simulink model "ex4_3"  (R2017a)
settings: Solver=ode23t  StartTime=0.0  StopTime=.3  MaxStep=1e-5  RelTol=1e-4  EnableMultiTasking=on
undefined symbols (not defined in the file): jsin
libraries: simulink x1, powerlib x1
settings Model: Creator=hi  LastModifiedBy=Omid
settings DataIOCC: LimitDataPoints=on
settings OptimizationCC: LifeSpan=inf
settings DebuggingCC: SFUnexpectedBacktrackingDiag=warning  SFNoUnconditionalDefaultTransitionDiag=warning  SFExecutionAtInitializationDiag=none
settings HardwareCC: ProdBitPerSizeT=32  ProdBitPerPtrDiffT=32  ProdWordSize=32  ProdHWDeviceType=Specified
settings ModelReferenceCC: PropagateSignalLabelsOutOfModel=off
settings GRTTargetCC: TargetLangStandard=C89/C90 (ANSI)
settings ConfigComp: CovMetricSettings=dw  CovSaveCumulativeToWorkspaceVar=on  CovSaveSingleToWorkspaceVar=on  CovExternalEMLEnable=off
settings SimscapeCC: SimscapeNormalizeSystem=off
settings ConfigurationSet: Description=SimMechanics 2G

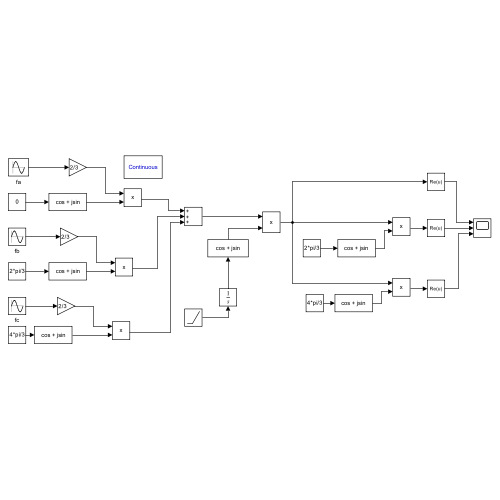
[thumbnail: Simulink's stored preview of the top-level diagram]
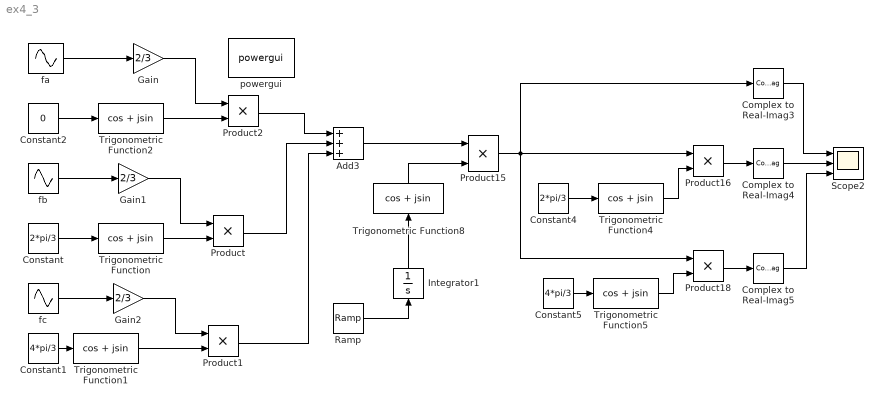
== system ex4_3 ==
  Add3 : Sum  Inputs=+++
  Complex to Real-Imag3 : ComplexToRealImag  Output=Real
  Complex to Real-Imag4 : ComplexToRealImag  Output=Real
  Complex to Real-Imag5 : ComplexToRealImag  Output=Real
  Constant : Constant  Value=2*pi/3
  Constant1 : Constant  Value=4*pi/3
  Constant2 : Constant  Value=0
  Constant4 : Constant  Value=2*pi/3
  Constant5 : Constant  Value=4*pi/3
  Gain : Gain  Gain=2/3
  Gain1 : Gain  Gain=2/3
  Gain2 : Gain  Gain=2/3
  Integrator1 : Integrator
  Product{,1..2,15..16,18} (6 alike) : Product
  Ramp : simulink/Sources/Ramp  slope=-2*pi*400  start=0  X0=0
  Scope2 : Scope  NumInputPorts=3
  Trigonometric Function{,1..2,4..5,8} (6 alike) : Trigonometry  Operator=cos + jsin
  fa : Sin  Frequency=377  Phase=pi/2  SampleTime=0
  fb : Sin  Frequency=377  Phase=-2*pi/3+pi/2  SampleTime=0
  fc : Sin  Frequency=377  Phase=-4*pi/3+pi/2  SampleTime=0
  powergui : powerlib/powergui  Priority=1  SimulationMode=Continuous  SampleTime=50e-6  frequency=60  Iterations=50  frequencyindice=60  Pbase=100e6  ErrMax=1e-4  UnitsV=kV  UnitsW=MW  buscounter=0  FunctionMessages=off  echomessages=off  EnableUseOfTLC=off  CurrentSourceSwitches=on  DisableSnubberDevices=off  DisableRonSwitches=off  DisableVfSwitches=off  DisplayEquations=off  AutomaticDiscreteSolvers=off  SolverType=Tustin/Backward Euler (TBE)  Interpol=off  ExternalGateDelay=off  methode=off  Ts=10  x0status=blocks  SPID=off  SwTol=0  HookPort=off  NonlinearTolerance=1e-4  nMaxIteration=100  ContinueOnMaxIteration=off  RestoreLinks=warning  ResistiveCurrentMeasurement=off  Frange=[0:2:500]  Ylog=off  Xlog=on  ShowGrid=off  save=off  variable=ZData  structure=0  ZoomFFT=off  StartTime=0.0  cycles=1  DisplayStyle=1  fundamental=60  FreqAxis=off  MaxFrequency=1000  frequencyindicesteady=1  RmsSteady=1  display=off
  wires:
  Constant/1 -> Trigonometric Function/1
  Trigonometric Function/1 -> Product/2
  Trigonometric Function1/1 -> Product1/2
  Constant1/1 -> Trigonometric Function1/1
  fc/1 -> Gain2/1
  fb/1 -> Gain1/1
  Constant2/1 -> Trigonometric Function2/1
  Trigonometric Function2/1 -> Product2/2
  fa/1 -> Gain/1
  Product2/1 -> Add3/1
  Product/1 -> Add3/2
  Product1/1 -> Add3/3
  Add3/1 -> Product15/1
  Constant4/1 -> Trigonometric Function4/1
  Constant5/1 -> Trigonometric Function5/1
  Product15/1 -> Complex to Real-Imag3/1, Product16/1, Product18/1
  Trigonometric Function4/1 -> Product16/2
  Trigonometric Function5/1 -> Product18/2
  Product16/1 -> Complex to Real-Imag4/1
  Product18/1 -> Complex to Real-Imag5/1
  Complex to Real-Imag4/1 -> Scope2/2
  Complex to Real-Imag3/1 -> Scope2/1
  Complex to Real-Imag5/1 -> Scope2/3
  Gain/1 -> Product2/1
  Gain1/1 -> Product/1
  Gain2/1 -> Product1/1
  Trigonometric Function8/1 -> Product15/2
  Integrator1/1 -> Trigonometric Function8/1
  Ramp/1 -> Integrator1/1
